simulink model "System"  (R2020b)
settings: Solver=VariableStepAuto  StartTime=0.0  StopTime=10.0  RelTol=1e-3
libraries: powerlib x7, spsFuelCellStackLib x1, powerlib_meascontrol x1
settings Model: Creator=Abdelhak_Samir  LastModifiedBy=Abdelhak_Samir
settings DebuggingCC: UnconnectedInputMsg=none  UnconnectedOutputMsg=none  UnconnectedLineMsg=none
settings ModelReferenceCC: EnableRefExpFcnMdlSchedulingChecks=off
settings RTWCC: GPUComputeCapability=5.0
settings ConfigComp: CovBoundaryAbsTol=1.0e-5

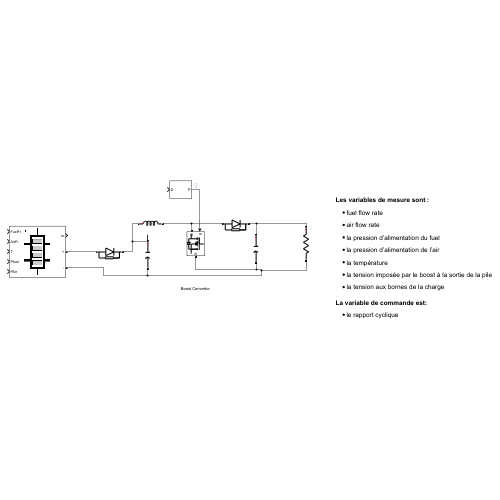
[thumbnail: Simulink's stored preview of the top-level diagram]
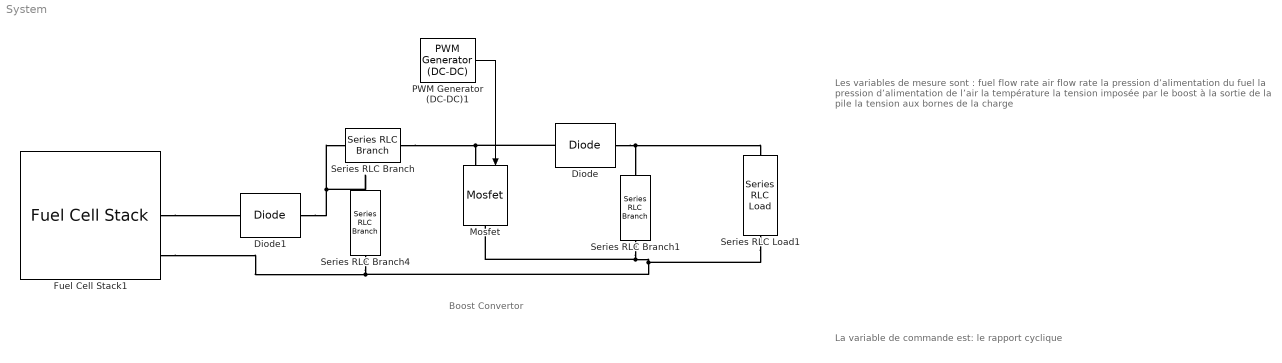
== system System ==
  note: Les variables de mesure sont :
      | fuel flow rate
      | air flow rate
      | la pression d’alimentation du fuel
      | la pression d’alimentation de l’air
      | la température
      | la tension imposée par le boost à la sortie de la pile
      | la tension aux bornes de la charge
  note: Boost Convertor
  note: La variable de commande est:
      | le rapport cyclique
  Diode : powerlib/Power Electronics/Diode  Ron=0.001  Lon=0  Vf=0.7  IC=0  UseSnubber=0  Rs=500  Cs=250e-9  Measurements=off
  Diode1 : powerlib/Power Electronics/Diode  Ron=0.001  Lon=0  Vf=0.7  IC=0  UseSnubber=0  Rs=500  Cs=250e-9  Measurements=off
  Fuel Cell Stack1 : spsFuelCellStackLib/Fuel Cell Stack  PresetModel=PEMFC - 1.26 kW - 24 Vdc  FcType=0  Detailed=Detailed  Eoc=[42,35]  NomVI=[52,24.23]  EndVI=[100,20]  Nc=42  n=46  TOp=55  AirFr=2400  SuppPress=[1.5,1]  Comp=[99.95,21,1]  SignX=off  SignY=off  FlowRateH2=on  FlowRateAir=on  SystemTemp=on  SystemPH2=on  SystemPAir=on  FCDyn=off  FC_tau=1  Peak_O2=80  V_Under=10
  Mosfet : powerlib/Power Electronics/Mosfet  Ron=0.1  Lon=0  Rd=0.01  Vfd=0.7  IC=0  Rs=1e5  Cs=10^-9  Measurements=off
  PWM Generator (DC-DC)1 : powerlib_meascontrol/Pulse & Signal Generators/PWM Generator (DC-DC)  Fsw=10000  Ts=0
  Series RLC Branch : powerlib/Elements/Series RLC Branch  LConnTagsString=__new0  RConnTagsString=__new0  BranchType=L  Resistance=1  Inductance=1e-4  SetiL0=off  InitialCurrent=0  Capacitance=1e-6  Setx0=off  InitialVoltage=0  Measurements=None
  Series RLC Branch1 : powerlib/Elements/Series RLC Branch  LConnTagsString=__new0  RConnTagsString=__new0  BranchType=C  Resistance=1  Inductance=1e-4  SetiL0=off  InitialCurrent=0  Capacitance=4700e-6  Setx0=off  InitialVoltage=0  Measurements=None
  Series RLC Branch4 : powerlib/Elements/Series RLC Branch  LConnTagsString=__new0  RConnTagsString=__new0  BranchType=C  Resistance=1  Inductance=1e-4  SetiL0=off  InitialCurrent=0  Capacitance=4700e-5  Setx0=on  InitialVoltage=42  Measurements=None
  Series RLC Load1 : powerlib/Elements/Series RLC Load  LConnTagsString=a  RConnTagsString=__new0  NominalVoltage=50  NominalFrequency=500  ActivePower=33  InductivePower=0  CapacitivePower=0  Setx0=off  InitialVoltage=0  SetiL0=off  InitialCurrent=0  Measurements=None  LoadType=constant Z
  wires:
  PWM Generator (DC-DC)1/1 -> Mosfet/1
  connections:
  Diode1/RConn1 -- Series RLC Branch4/LConn1 -- Series RLC Branch/LConn1
  Series RLC Branch1/RConn1 -- Series RLC Load1/RConn1 -- Fuel Cell Stack1/RConn2 -- Series RLC Branch4/RConn1 -- Mosfet/RConn1
  Series RLC Branch/RConn1 -- Diode/LConn1 -- Mosfet/LConn1
  Diode/RConn1 -- Series RLC Load1/LConn1 -- Series RLC Branch1/LConn1
  Fuel Cell Stack1/RConn1 -- Diode1/LConn1
